simulink model "TempomatV1"  (R2018b)
settings: Solver=FixedStepAuto  StartTime=0.0  StopTime=100.0  FixedStep=0.001  RelTol=1e-3
settings Model: Creator=marci  LastModifiedBy=marci

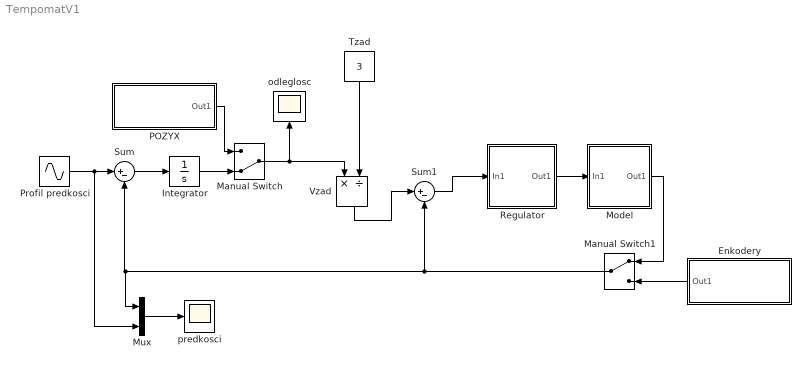
== system TempomatV1 ==
  Enkodery : Subsystem
  Integrator : Integrator  InitialCondition=3
  Manual Switch : ManualSwitch  CurrentSetting=0
  Manual Switch1 : ManualSwitch
  Model : Subsystem
  Mux : Mux  Inputs=2
  POZYX : Subsystem
  Profil predkosci : Sin  Amplitude=0.5  Bias=3  Frequency=0.5  SampleTime=0
  Regulator : Subsystem
  Sum : Sum  Inputs=|+-
  Sum1 : Sum  Inputs=|+-
  Tzad : Constant  Value=3
  Vzad : Product  Inputs=*/
  "odleglosc " : Scope
  predkosci : Scope
  wires:
  Sum/1 -> Integrator/1
  Tzad/1 -> Vzad/2
  Vzad/1 -> Sum1/1
  Mux/1 -> predkosci/1
  Sum1/1 -> Regulator/1(In1)
  Regulator/1(Out1) -> Model/1(In1)
  Model/1(Out1) -> Manual Switch1/1
  Manual Switch1/1 -> Sum1/2, Sum/2, Mux/1
  Integrator/1 -> Manual Switch/2
  POZYX/1(Out1) -> Manual Switch/1
  Profil predkosci/1 -> Mux/2, Sum/1
  Manual Switch/1 -> Vzad/1, "odleglosc "/1
  Enkodery/1(Out1) -> Manual Switch1/2

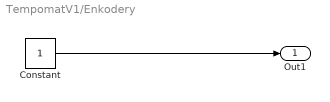
== system TempomatV1/Enkodery ==
  Constant : Constant
  Out1 : Outport
  wires:
  Constant/1 -> Out1/1

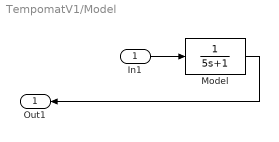
== system TempomatV1/Model ==
  In1 : Inport
  Model : TransferFcn  Denominator=[5 1]
  Out1 : Outport
  wires:
  In1/1 -> Model/1
  Model/1 -> Out1/1

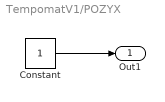
== system TempomatV1/POZYX ==
  Constant : Constant
  Out1 : Outport
  wires:
  Constant/1 -> Out1/1

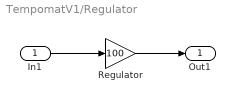
== system TempomatV1/Regulator ==
  In1 : Inport
  Regulator : Gain  Gain=100
  Out1 : Outport
  wires:
  Regulator/1 -> Out1/1
  In1/1 -> Regulator/1
